simulink model "quarter_sus_imp_force"  (R2025a)
settings: Solver=FixedStepAuto  StartTime=0.0  StopTime=20  FixedStep=0.001  RelTol=1e-3
model workspace (MAT data in the model file):
  Cs : Simulink.Parameter (value not decoded)
  Cy_f1 = 128915.5
  Cy_r1 = 85943.6
  G0 : Simulink.Parameter (value not decoded)
  IDA_ISD_PBC_bd : Simulink.Parameter (value not decoded)
  IDA_ISD_PBC_c1 : Simulink.Parameter (value not decoded)
  IDA_ISD_PBC_k1 : Simulink.Parameter (value not decoded)
  IDA_ISD_PBC_k2 : Simulink.Parameter (value not decoded)
  IDA_ISD_PBC_r1 : Simulink.Parameter (value not decoded)
  IDA_PBC_cd4 = 2000
  IDA_PBC_kd2 = 10000
  IDA_PBC_r1 = 1.5
  IDA_PBC_r2 = 0.44
  ISD_1_b : Simulink.Parameter (value not decoded)
  ISD_1_c : Simulink.Parameter (value not decoded)
  ISD_1_k1 : Simulink.Parameter (value not decoded)
  ISD_1_k2 : Simulink.Parameter (value not decoded)
  Izz1 = 1536.7
  Ks : Simulink.Parameter (value not decoded)
  Kt : Simulink.Parameter (value not decoded)
  Q : Simulink.Parameter (value not decoded)
  Q_F : Simulink.Parameter (value not decoded)
  Q_b_deflec : Simulink.Parameter (value not decoded)
  Q_delta_F : Simulink.Parameter (value not decoded)
  Q_dot : Simulink.Parameter (value not decoded)
  Q_dot_s : Simulink.Parameter (value not decoded)
  Q_dot_s_h : Simulink.Parameter (value not decoded)
  Q_dot_u : Simulink.Parameter (value not decoded)
  Q_flec : Simulink.Parameter (value not decoded)
  Q_flec_t : Simulink.Parameter (value not decoded)
  SHADD_alpha : Simulink.Parameter (value not decoded)
  a1 = 1.015
  a_max : Simulink.Parameter (value not decoded)
  a_min : Simulink.Parameter (value not decoded)
  adva_max : Simulink.Parameter (value not decoded)
  adva_min : Simulink.Parameter (value not decoded)
  as_max : Simulink.Parameter (value not decoded)
  b1 = 1.895
  b_deflec : Simulink.Parameter (value not decoded)
  bump_height : Simulink.Parameter (value not decoded)
  bump_lenth : Simulink.Parameter (value not decoded)
  bump_start : Simulink.Parameter (value not decoded)
  damper_param : Simulink.Parameter (value not decoded)
  deflec_max : Simulink.Parameter (value not decoded)
  done_range : Simulink.Parameter (value not decoded)
  f0 : Simulink.Parameter (value not decoded)
  h1 = 0.54
  imp_Cs : Simulink.Parameter (value not decoded)
  imp_Ks : Simulink.Parameter (value not decoded)
  imp_Ms : Simulink.Parameter (value not decoded)
  inerter_b : Simulink.Parameter (value not decoded)
  inerter_b_2 : Simulink.Parameter (value not decoded)
  inerter_c : Simulink.Parameter (value not decoded)
  inerter_k : Simulink.Parameter (value not decoded)
  inerter_k_2 : Simulink.Parameter (value not decoded)
  ms : Simulink.Parameter (value not decoded)
  mu : Simulink.Parameter (value not decoded)
  noise_seed : Simulink.Parameter (value not decoded)
  omega_1 : Simulink.Parameter (value not decoded)
  omega_2 : Simulink.Parameter (value not decoded)
  omega_3 : Simulink.Parameter (value not decoded)
  omega_4 : Simulink.Parameter (value not decoded)
  omega_5 : Simulink.Parameter (value not decoded)
  punish_Q : Simulink.Parameter (value not decoded)
  punish_R : Simulink.Parameter (value not decoded)
  reward_w_as : Simulink.Parameter (value not decoded)
  reward_w_au : Simulink.Parameter (value not decoded)
  reward_w_defv : Simulink.Parameter (value not decoded)
  road_seed : Simulink.Parameter (value not decoded)
  road_type : Simulink.Parameter (value not decoded)
  sigma_f1 = 0.1
  sigma_r1 = 0.1
  sine_amp : Simulink.Parameter (value not decoded)
  sine_freq : Simulink.Parameter (value not decoded)
  u : Simulink.Parameter (value not decoded)
  vs0 : Simulink.Parameter (value not decoded)
  vu0 : Simulink.Parameter (value not decoded)
  x_max : Simulink.Parameter (value not decoded)
  x_min : Simulink.Parameter (value not decoded)
  xs0 : Simulink.Parameter (value not decoded)
  xu0 : Simulink.Parameter (value not decoded)
symbols that are objects in the model workspace (value not decoded): a_max, a_min, b_deflec, bump_height, bump_lenth, bump_start, Cs, damper_param, f0, G0, IDA_ISD_PBC_bd, IDA_ISD_PBC_c1, IDA_ISD_PBC_k1, IDA_ISD_PBC_k2, IDA_ISD_PBC_r1, imp_Cs, imp_Ks, imp_Ms, Ks, Kt, ms, mu, omega_1, omega_2, omega_3, omega_4, omega_5, Q_b_deflec, Q_delta_F, Q_dot_s, Q_dot_s_h, Q_dot_u, Q_F, Q_flec, Q_flec_t, road_type, SHADD_alpha, sine_amp, sine_freq, vs0, vu0, xs0, xu0
undefined symbols (not defined in the file): ADD, Force, IDA, Imp, Imp_Force, PBC, SH, Train, Validation
libraries: fl_lib x32, nesl_utility x27, sharedTrackingLibrary x4, sdl_lib x2, dspstat3 x2, deeplib x1, simulink x1
(part 6 of 6)

== system quarter_sus_imp_force/QuarterSuspension /Variant Subsystem/Train-Imp_Force/Subsystem/MATLAB Function2/EKF epsilon ==
  y : Inport
  epsilon : Inport  Port=2
  Constant : Constant  Value=diag([0,0,1,0])
  Constant7 : Constant  Value=500  SampleTime=0.001
  Extended Kalman Filter1 : sharedTrackingLibrary/Extended Kalman Filter  StateTransitionFcn=IFEKF_tfcn_ep  HasStateTransitionJacobianFcn=on  StateTransitionJacobianFcn=IFEKF_jcob_fcn_ep  HasAdditiveProcessNoise=Additive  ProcessNoise=[0,0,1e-7,1e-10]  HasTimeVaryingProcessNoise=on  HasStateTransitionFcnExtraArgument=1  InitialState=[0;-0.2;1*2*pi;0.2;]  InitialStateCovariance=[1e-1,1e-1,1e-1,1e-5]  MeasurementFcn1=IFEKF_measure_fcn_mod  HasMeasurementJacobianFcn1=on  MeasurementJacobianFcn1=IFEKF_mea_jcob_fcn_mod  HasMeasurementEnablePort1=off  HasAdditiveMeasurementNoise1=Additive  MeasurementNoise1=0.0001  HasTimeVaryingMeasurementNoise1=on  HasMeasurementFcnExtraArgument1=0  HasMeasurementWrapping1=off  MeasurementFcn2=myMeasurementFcn  HasMeasurementJacobianFcn2=off  HasMeasurementEnablePort2=off  HasAdditiveMeasurementNoise2=Additive  MeasurementNoise2=1  HasTimeVaryingMeasurementNoise2=off  HasMeasurementFcnExtraArgument2=0  HasMeasurementWrapping2=off  MeasurementFcn3=myMeasurementFcn  HasMeasurementJacobianFcn3=off  HasMeasurementEnablePort3=off  HasAdditiveMeasurementNoise3=Additive  MeasurementNoise3=1  HasTimeVaryingMeasurementNoise3=off  HasMeasurementFcnExtraArgument3=0  HasMeasurementWrapping3=off  MeasurementFcn4=myMeasurementFcn  HasMeasurementJacobianFcn4=off  HasMeasurementEnablePort4=off  HasAdditiveMeasurementNoise4=Additive  MeasurementNoise4=1  HasTimeVaryingMeasurementNoise4=off  HasMeasurementFcnExtraArgument4=0  HasMeasurementWrapping4=off  MeasurementFcn5=myMeasurementFcn  HasMeasurementJacobianFcn5=off  HasMeasurementEnablePort5=off  HasAdditiveMeasurementNoise5=Additive  MeasurementNoise5=1  HasTimeVaryingMeasurementNoise5=off  HasMeasurementFcnExtraArgument5=0  HasMeasurementWrapping5=off  EnableMultirate=off  StateTransitionFcnSampleTime=1  MeasurementFcn1SampleTime=1  MeasurementFcn2SampleTime=1  MeasurementFcn3SampleTime=1  MeasurementFcn4SampleTime=1  MeasurementFcn5SampleTime=1  UseCurrentEstimator=off  OutputStateCovariance=on  DataType=double  SampleTime=0.001  NumberOfMeasurements=1
  Gain6 : Gain  Gain=1/2/pi
  Scope6 : Scope
      settings: ActiveDisplayYMinimum=-0.3996  ActiveDisplayYMaximum=6.537  DataLoggingVariableName=ScopeData2
  Selector1 : Selector  InputPortWidth=4  IndexOptions=Index vector (dialog)  Indices=[1]  OutputSizes=1
  Selector8 : Selector  InputPortWidth=4  IndexOptions=Index vector (dialog)  Indices=[3]  OutputSizes=1
  x1hat : Outport
  P : Outport  Port=2
  debug : Outport  Port=3
  xhat_pred : Outport  Port=4
  y_residual : Outport  Port=5
  omega : Outport  Port=6
  wires:
  y/1 -> Extended Kalman Filter1/3
  Extended Kalman Filter1/2 -> P/1
  Constant7/1 -> Extended Kalman Filter1/4
  epsilon/1 -> Extended Kalman Filter1/2
  Constant/1 -> Extended Kalman Filter1/1
  Gain6/1 -> omega/1, Scope6/1
  Selector8/1 -> Gain6/1
  Extended Kalman Filter1/1 -> Selector1/1, Selector8/1
  Selector1/1 -> x1hat/1

== system quarter_sus_imp_force/QuarterSuspension /Variant Subsystem/Train-Imp_Force/Subsystem/MATLAB Function2/EKF simple Amp ==
  y : Inport
  epsilon : Inport  Port=2
  Constant5 : Constant  Value=0.1e-5
  Constant7 : Constant  Value=0.11  SampleTime=0.001
  Extended Kalman Filter1 : sharedTrackingLibrary/Extended Kalman Filter  StateTransitionFcn=IFEKF_tfcn_amp  HasStateTransitionJacobianFcn=on  StateTransitionJacobianFcn=IFEKF_jcob_fcn_amp  HasAdditiveProcessNoise=Additive  ProcessNoise=[0,0,1e-7,1e-10]  HasTimeVaryingProcessNoise=on  HasStateTransitionFcnExtraArgument=1  InitialState=[0;-0.5;2*pi;0.5;]  InitialStateCovariance=[1e-1,1e-1,1e-1,1e-5]  MeasurementFcn1=IFEKF_measure_fcn_amp  HasMeasurementJacobianFcn1=on  MeasurementJacobianFcn1=IFEKF_mea_jcob_fcn_amp  HasMeasurementEnablePort1=off  HasAdditiveMeasurementNoise1=Additive  MeasurementNoise1=0.0001  HasTimeVaryingMeasurementNoise1=on  HasMeasurementFcnExtraArgument1=0  HasMeasurementWrapping1=off  MeasurementFcn2=myMeasurementFcn  HasMeasurementJacobianFcn2=off  HasMeasurementEnablePort2=off  HasAdditiveMeasurementNoise2=Additive  MeasurementNoise2=1  HasTimeVaryingMeasurementNoise2=off  HasMeasurementFcnExtraArgument2=0  HasMeasurementWrapping2=off  MeasurementFcn3=myMeasurementFcn  HasMeasurementJacobianFcn3=off  HasMeasurementEnablePort3=off  HasAdditiveMeasurementNoise3=Additive  MeasurementNoise3=1  HasTimeVaryingMeasurementNoise3=off  HasMeasurementFcnExtraArgument3=0  HasMeasurementWrapping3=off  MeasurementFcn4=myMeasurementFcn  HasMeasurementJacobianFcn4=off  HasMeasurementEnablePort4=off  HasAdditiveMeasurementNoise4=Additive  MeasurementNoise4=1  HasTimeVaryingMeasurementNoise4=off  HasMeasurementFcnExtraArgument4=0  HasMeasurementWrapping4=off  MeasurementFcn5=myMeasurementFcn  HasMeasurementJacobianFcn5=off  HasMeasurementEnablePort5=off  HasAdditiveMeasurementNoise5=Additive  MeasurementNoise5=1  HasTimeVaryingMeasurementNoise5=off  HasMeasurementFcnExtraArgument5=0  HasMeasurementWrapping5=off  EnableMultirate=off  StateTransitionFcnSampleTime=1  MeasurementFcn1SampleTime=1  MeasurementFcn2SampleTime=1  MeasurementFcn3SampleTime=1  MeasurementFcn4SampleTime=1  MeasurementFcn5SampleTime=1  UseCurrentEstimator=off  OutputStateCovariance=on  DataType=double  SampleTime=0.001  NumberOfMeasurements=1
  Gain6 : Gain  Gain=1/2/pi
  MATLAB Function : MATLAB Function
  Scope1 : Scope
      settings: ActiveDisplayYMinimum=-1.3479  ActiveDisplayYMaximum=7.1311  DataLoggingVariableName=ScopeData7
  Scope6 : Scope
      settings: ActiveDisplayYMinimum=0.95  ActiveDisplayYMaximum=1.05
  Selector1 : Selector  InputPortWidth=4  IndexOptions=Index vector (dialog)  Indices=[1]  OutputSizes=1
  Selector8 : Selector  InputPortWidth=4  IndexOptions=Index vector (dialog)  Indices=[3]  OutputSizes=1
  x1hat : Outport
  P : Outport  Port=2
  debug : Outport  Port=3
  xhat_pred : Outport  Port=4
  y_residual : Outport  Port=5
  omega : Outport  Port=6
  wires:
  epsilon/1 -> Extended Kalman Filter1/2
  Constant7/1 -> Extended Kalman Filter1/4
  Constant5/1 -> MATLAB Function/1(gamma)
  Extended Kalman Filter1/2 -> P/1
  y/1 -> Extended Kalman Filter1/3
  MATLAB Function/1(y) -> Extended Kalman Filter1/1
  Extended Kalman Filter1/1 -> Selector1/1, Selector8/1, Scope1/1
  Selector8/1 -> Gain6/1
  Gain6/1 -> omega/1, Scope6/1
  Selector1/1 -> x1hat/1

== system quarter_sus_imp_force/QuarterSuspension /Variant Subsystem/Train-Imp_Force/Subsystem/MATLAB Function2/IFEKF simple ==
  y : Inport
  Constant : Constant  Value=diag([0,0,0,0,1])
  Constant7 : Constant  Value=10  SampleTime=0.001
  Extended Kalman Filter1 : sharedTrackingLibrary/Extended Kalman Filter  StateTransitionFcn=IFEKF_tfcn_simp  HasStateTransitionJacobianFcn=on  StateTransitionJacobianFcn=IFEKF_jcob_fcn_simp  HasAdditiveProcessNoise=Additive  ProcessNoise=[0,0,1e-7,1e-10,0]  HasTimeVaryingProcessNoise=on  HasStateTransitionFcnExtraArgument=0  InitialState=[0;-1;0;-1;0.1*pi;]  InitialStateCovariance=[1e-1,1e-1,1e-1,1e-1,1e-5]  MeasurementFcn1=IFEKF_measure_fcn_simp  HasMeasurementJacobianFcn1=on  MeasurementJacobianFcn1=IFEKF_mea_jcob_fcn_simp  HasMeasurementEnablePort1=off  HasAdditiveMeasurementNoise1=Additive  MeasurementNoise1=0.0001  HasTimeVaryingMeasurementNoise1=on  HasMeasurementFcnExtraArgument1=0  HasMeasurementWrapping1=off  MeasurementFcn2=myMeasurementFcn  HasMeasurementJacobianFcn2=off  HasMeasurementEnablePort2=off  HasAdditiveMeasurementNoise2=Additive  MeasurementNoise2=1  HasTimeVaryingMeasurementNoise2=off  HasMeasurementFcnExtraArgument2=0  HasMeasurementWrapping2=off  MeasurementFcn3=myMeasurementFcn  HasMeasurementJacobianFcn3=off  HasMeasurementEnablePort3=off  HasAdditiveMeasurementNoise3=Additive  MeasurementNoise3=1  HasTimeVaryingMeasurementNoise3=off  HasMeasurementFcnExtraArgument3=0  HasMeasurementWrapping3=off  MeasurementFcn4=myMeasurementFcn  HasMeasurementJacobianFcn4=off  HasMeasurementEnablePort4=off  HasAdditiveMeasurementNoise4=Additive  MeasurementNoise4=1  HasTimeVaryingMeasurementNoise4=off  HasMeasurementFcnExtraArgument4=0  HasMeasurementWrapping4=off  MeasurementFcn5=myMeasurementFcn  HasMeasurementJacobianFcn5=off  HasMeasurementEnablePort5=off  HasAdditiveMeasurementNoise5=Additive  MeasurementNoise5=1  HasTimeVaryingMeasurementNoise5=off  HasMeasurementFcnExtraArgument5=0  HasMeasurementWrapping5=off  EnableMultirate=off  StateTransitionFcnSampleTime=1  MeasurementFcn1SampleTime=1  MeasurementFcn2SampleTime=1  MeasurementFcn3SampleTime=1  MeasurementFcn4SampleTime=1  MeasurementFcn5SampleTime=1  UseCurrentEstimator=off  OutputStateCovariance=on  DataType=double  SampleTime=0.001  NumberOfMeasurements=1
  Gain6 : Gain  Gain=1/2/pi
  Scope1 : Scope
      settings: ActiveDisplayYMinimum=-108223.313  ActiveDisplayYMaximum=120159.3313  DataLoggingVariableName=ScopeData2
  Scope6 : Scope
      settings: ActiveDisplayYMinimum=-5.0452  ActiveDisplayYMaximum=3.9569  DataLoggingVariableName=ScopeData3
  Selector1 : Selector  InputPortWidth=5  IndexOptions=Index vector (dialog)  Indices=[1]  OutputSizes=1
  Selector8 : Selector  InputPortWidth=5  IndexOptions=Index vector (dialog)  Indices=[5]  OutputSizes=1
  x1hat : Outport
  P : Outport  Port=2
  debug : Outport  Port=3
  xhat_pred : Outport  Port=4
  y_residual : Outport  Port=5
  omega : Outport  Port=6
  wires:
  y/1 -> Extended Kalman Filter1/2
  Extended Kalman Filter1/2 -> P/1
  Constant7/1 -> Extended Kalman Filter1/3
  Constant/1 -> Extended Kalman Filter1/1
  Gain6/1 -> omega/1, Scope6/1
  Selector8/1 -> Gain6/1
  Selector1/1 -> x1hat/1
  Extended Kalman Filter1/1 -> Selector1/1, Selector8/1, Scope1/1

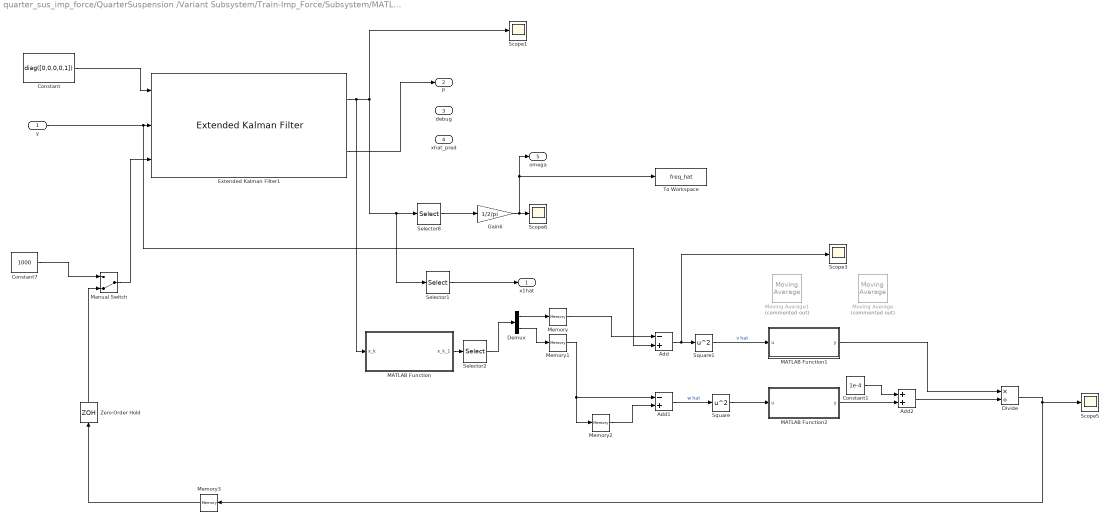
== system quarter_sus_imp_force/QuarterSuspension /Variant Subsystem/Train-Imp_Force/Subsystem/MATLAB Function2/adaptive IFEKF simple ==
  y : Inport
  Add : Sum  Inputs=-+
  Add1 : Sum  Inputs=-+
  Add2 : Sum
  Constant : Constant  Value=diag([0,0,0,0,1])
  Constant1 : Constant  Value=1e-4
  Constant7 : Constant  Value=1000  SampleTime=0.001
  Demux : Demux  Outputs=2
  Divide : Product  Inputs=*/
  Extended Kalman Filter1 : sharedTrackingLibrary/Extended Kalman Filter  StateTransitionFcn=IFEKF_tfcn_simp  HasStateTransitionJacobianFcn=on  StateTransitionJacobianFcn=IFEKF_jcob_fcn_simp  HasAdditiveProcessNoise=Additive  ProcessNoise=[0,0,1e-7,1e-10,0]  HasTimeVaryingProcessNoise=on  HasStateTransitionFcnExtraArgument=0  InitialState=[0;-1;0;-1;0.1*pi;]  InitialStateCovariance=[1e-1,1e-1,1e-1,1e-1,1e-5]  MeasurementFcn1=IFEKF_measure_fcn_simp  HasMeasurementJacobianFcn1=on  MeasurementJacobianFcn1=IFEKF_mea_jcob_fcn_simp  HasMeasurementEnablePort1=off  HasAdditiveMeasurementNoise1=Additive  MeasurementNoise1=0.0001  HasTimeVaryingMeasurementNoise1=on  HasMeasurementFcnExtraArgument1=0  HasMeasurementWrapping1=off  MeasurementFcn2=myMeasurementFcn  HasMeasurementJacobianFcn2=off  HasMeasurementEnablePort2=off  HasAdditiveMeasurementNoise2=Additive  MeasurementNoise2=1  HasTimeVaryingMeasurementNoise2=off  HasMeasurementFcnExtraArgument2=0  HasMeasurementWrapping2=off  MeasurementFcn3=myMeasurementFcn  HasMeasurementJacobianFcn3=off  HasMeasurementEnablePort3=off  HasAdditiveMeasurementNoise3=Additive  MeasurementNoise3=1  HasTimeVaryingMeasurementNoise3=off  HasMeasurementFcnExtraArgument3=0  HasMeasurementWrapping3=off  MeasurementFcn4=myMeasurementFcn  HasMeasurementJacobianFcn4=off  HasMeasurementEnablePort4=off  HasAdditiveMeasurementNoise4=Additive  MeasurementNoise4=1  HasTimeVaryingMeasurementNoise4=off  HasMeasurementFcnExtraArgument4=0  HasMeasurementWrapping4=off  MeasurementFcn5=myMeasurementFcn  HasMeasurementJacobianFcn5=off  HasMeasurementEnablePort5=off  HasAdditiveMeasurementNoise5=Additive  MeasurementNoise5=1  HasTimeVaryingMeasurementNoise5=off  HasMeasurementFcnExtraArgument5=0  HasMeasurementWrapping5=off  EnableMultirate=off  StateTransitionFcnSampleTime=1  MeasurementFcn1SampleTime=1  MeasurementFcn2SampleTime=1  MeasurementFcn3SampleTime=1  MeasurementFcn4SampleTime=1  MeasurementFcn5SampleTime=1  UseCurrentEstimator=off  OutputStateCovariance=on  DataType=double  SampleTime=0.001  NumberOfMeasurements=1
  Gain6 : Gain  Gain=1/2/pi
  MATLAB Function : MATLAB Function  TreatAsAtomicUnit=on
  MATLAB Function1 : MATLAB Function  TreatAsAtomicUnit=on
  MATLAB Function2 : MATLAB Function  TreatAsAtomicUnit=on
  Manual Switch : ManualSwitch  CurrentSetting=0
  Memory : Memory  InitialCondition=5
  Memory1 : Memory
  Memory2 : Memory  InitialCondition=1
  Memory3 : Memory  InitialCondition=10
  Moving Average : dspstat3/Moving Average  Commented=on  Method=Exponential weighting  ForgettingFactorPort=off  SpecifyWindowLength=off  WindowLength=100  OverlapLength=50  AllowArbitraryInputLength=on  ForgettingFactor=0.999  SimulateUsing=Interpreted execution
  Moving Average1 : dspstat3/Moving Average  Commented=on  Method=Sliding window  ForgettingFactorPort=off  SpecifyWindowLength=off  WindowLength=100  OverlapLength=50  AllowArbitraryInputLength=off  ForgettingFactor=0.999  SimulateUsing=Code generation
  Scope{1,3,5..6} (4 alike) : Scope
      Scope1 settings: ActiveDisplayYMinimum=-5.9836760801118811E+37  ActiveDisplayYMaximum=5.3206752918754988E+37  DataLoggingVariableName=ScopeData3
      Scope3 settings: ActiveDisplayYMinimum=-5.9322  ActiveDisplayYMaximum=3.4471  DataLoggingVariableName=ScopeData4
      Scope5 settings: ActiveDisplayYMinimum=-182.5988  ActiveDisplayYMaximum=1643.3904  DataLoggingVariableName=ScopeData6
      Scope6 settings: ActiveDisplayYMinimum=-3.1891  ActiveDisplayYMaximum=3.1646  DataLoggingVariableName=ScopeData8
  Selector1 : Selector  InputPortWidth=5  IndexOptions=Index vector (dialog)  Indices=[1]  OutputSizes=1
  Selector2 : Selector  InputPortWidth=5  IndexOptions=Index vector (dialog)  Indices=[1 5]  OutputSizes=1
  Selector8 : Selector  InputPortWidth=5  IndexOptions=Index vector (dialog)  Indices=[5]  OutputSizes=1
  Square : Math  Operator=square
  Square1 : Math  Operator=square
  To Workspace : ToWorkspace  VariableName=freq_hat  SampleTime=-1
  Zero-Order Hold : ZeroOrderHold  SampleTime=0.001
  x1hat : Outport
  P : Outport  Port=2
  debug : Outport  Port=3
  xhat_pred : Outport  Port=4
  omega : Outport  Port=5
  wires:
  Add1/1 -> Square/1  "w hat"
  Demux/2 -> Memory1/1
  Constant1/1 -> Add2/1
  Zero-Order Hold/1 -> Manual Switch/2
  Memory2/1 -> Add1/2
  Manual Switch/1 -> Extended Kalman Filter1/3
  MATLAB Function/1(x_k_1) -> Selector2/1
  MATLAB Function1/1(y) -> Divide/1
  Selector2/1 -> Demux/1
  Add2/1 -> Divide/2
  Constant/1 -> Extended Kalman Filter1/1
  Selector1/1 -> x1hat/1
  MATLAB Function2/1(y) -> Add2/2
  Memory/1 -> Add/1
  Extended Kalman Filter1/1 -> MATLAB Function/1(x_k), Scope1/1, Selector8/1, Selector1/1
  y/1 -> Add/2, Extended Kalman Filter1/2
  Memory1/1 -> Add1/1, Memory2/1
  Square/1 -> MATLAB Function2/1(u)
  Square1/1 -> MATLAB Function1/1(u)  "v hat"
  Extended Kalman Filter1/2 -> P/1
  Divide/1 -> Memory3/1, Scope5/1
  Selector8/1 -> Gain6/1
  Demux/1 -> Memory/1
  Add/1 -> Scope3/1, Square1/1
  Memory3/1 -> Zero-Order Hold/1
  Gain6/1 -> Scope6/1, To Workspace/1, omega/1
  Constant7/1 -> Manual Switch/1

== matlab function quarter_sus_imp_force/QuarterSuspension /Variant Subsystem/IDA-PBC/Subsystem/我的控制/MATLAB Function ==
  data: cs input; ks input; ct input; r1 input; u output; r2 input; kd2 input; cd4 input; q1 input; q2 input; dq1 input; dq2 input
function u = calculateEquation(cs, ks,ct, r1, r2, kd2,cd4, q1,q2,dq1,dq2)
    % Calculate each term of the equation
    term1 = (ks - r2*kd2)*q1;
    term2 = (r1 - r2)*kd2*q2 + cs*dq1;
    % term4 = r2 * (r2 - r1)* cd4;
    term3 = (cd4/2 - cd4/r2 + (2*cd4)/(-r1 + r2)+cs)*dq1;
    
    term5 = (cd4/2 - (cd4*r1)/(2*r2)) * dq2;

    % Sum all terms to get u
    u = term1 + term2 + term3 - term5;
end

== matlab function quarter_sus_imp_force/QuarterSuspension /Variant Subsystem/PDD/Subsystem1/MATLAB Function ==
  data: Kxsvs input; y output; cmax input; cmin input; vdef input; xdef input; Cs input
function y = PDD_switch(Kxsvs,cmax,cmin,vdef, xdef,Cs)
vdef2 = vdef^2;
    if (Kxsvs + ((cmax + Cs) * vdef2)) < 0
        y = 1;
    elseif (vdef == 0) && (xdef ~= 0) 
        y = 3;
    elseif (Kxsvs + ((cmin +Cs) *vdef2)) >= 0
        y = 2;
    else
        y = 4 ;
    end
end

== matlab function quarter_sus_imp_force/QuarterSuspension /Variant Subsystem/IDA-PBC/Subsystem/IDA-PBC 论文控制/MATLAB Function ==
  data: cs input; ks input; ct input; r1 input; u output; r2 input; kd2 input; cd4 input; q1 input; q2 input; dq1 input; dq2 input
function u = calculateEquation(cs, ks,ct, r1, r2, kd2,cd4, q1,q2,dq1,dq2)
    % Calculate each term of the equation
    term1 = (ks - r2*kd2)*q1;
    term2 = (r1 - r2)*kd2*q2 + cs*dq1;
    term4 = r2 * (r2 - r1)* cd4;
    term3 = ((r1*r2*(r2 - 2)*ct +term4)*dq1) / (r1 - r2)^2;
    
    term5 = (ct*r1*r2 / (r1 - r2) - cd4) * dq2;

    % Sum all terms to get u
    u = term1 + term2 + term3 - term5;
end

== matlab function quarter_sus_imp_force/QuarterSuspension /Subsystem1/Semi Active Suspension/Damper/Hysteretic/MATLAB Function1 ==
  data: displacement input; F_d output; velocity input; I input; params input
function F_d = improvedHystereticModel(displacement, velocity, I, params)
    % 从params数组中提取模型参数
    c1 = params(1); c2 = params(2); c3 = params(3);
    k1 = params(4); k2 = params(5); k3 = params(6);
    alpha1 = params(7); alpha2 = params(8);
    % f01 = params(9); f02 = params(10); f03 = params(11); % 这些参数似乎在模型中未使用
    gamma1 = params(12); gamma2 = params(13); gamma3 = params(14);
    beta = params(15); delta = params(16);

    % 根据I计算c, k, alpha, 和 gamma
    c = c1 * I^2 + c2 * I + c3;
    k = k1 * I^2 + k2 * I + k3;
    alpha = alpha1 * I + alpha2;
    gamma = gamma1 * I^2 + gamma2 * I + gamma3;

    % 计算c^*和z
    c_star = gamma * (sign(velocity) + 1);
    z = tanh(beta * velocity + delta * sign(displacement));

    % 计算减震器力
    F_d = (c + c_star) * velocity + k * displacement + alpha * z;
end

== matlab function quarter_sus_imp_force/QuarterSuspension /Subsystem1/Semi Active Suspension/Damper/Random Current/MATLAB Function1 ==
  data: displacement input; F_d output; velocity input; I input; params input
function F_d = improvedHystereticModel(displacement, velocity, I, params)
    % 从params数组中提取模型参数
    c1 = params(1); c2 = params(2); c3 = params(3);
    k1 = params(4); k2 = params(5); k3 = params(6);
    alpha1 = params(7); alpha2 = params(8);
    % f01 = params(9); f02 = params(10); f03 = params(11); % 这些参数似乎在模型中未使用
    gamma1 = params(12); gamma2 = params(13); gamma3 = params(14);
    beta = params(15); delta = params(16);

    % 根据I计算c, k, alpha, 和 gamma
    c = c1 * I^2 + c2 * I + c3;
    k = k1 * I^2 + k2 * I + k3;
    alpha = alpha1 * I + alpha2;
    gamma = gamma1 * I^2 + gamma2 * I + gamma3;

    % 计算c^*和z
    c_star = gamma * (sign(velocity) + 1);
    z = tanh(beta * velocity + delta * sign(displacement));

    % 计算减震器力
    F_d = (c + c_star) * velocity + k * displacement + alpha * z;
end

== matlab function quarter_sus_imp_force/QuarterSuspension /Subsystem1/Semi Active Suspension/Damper/semi-active/MATLAB Function1 ==
  data: displacement input; F_d output; velocity input; I input; params input
function F_d = improvedHystereticModel(displacement, velocity, I, params)
    % 从params数组中提取模型参数
    c1 = params(1); c2 = params(2); c3 = params(3);
    k1 = params(4); k2 = params(5); k3 = params(6);
    alpha1 = params(7); alpha2 = params(8);
    % f01 = params(9); f02 = params(10); f03 = params(11); % 这些参数似乎在模型中未使用
    gamma1 = params(12); gamma2 = params(13); gamma3 = params(14);
    beta = params(15); delta = params(16);

    % 根据I计算c, k, alpha, 和 gamma
    c = c1 * I^2 + c2 * I + c3;
    k = k1 * I^2 + k2 * I + k3;
    alpha = alpha1 * I + alpha2;
    gamma = gamma1 * I^2 + gamma2 * I + gamma3;

    % 计算c^*和z
    c_star = gamma * (sign(velocity) + 1);
    z = tanh(beta * velocity + delta * sign(displacement));

    % 计算减震器力
    F_d = (c + c_star) * velocity + k * displacement + alpha * z;
end

== matlab function quarter_sus_imp_force/QuarterSuspension /Variant Subsystem/IDA-PBC/Subsystem/IDA_ISD_1号参考控制/MATLAB Function ==
  data: cs input; ks input; ct input; r1 input; u output; r2 input; k1 input; k2 input; c1 input; q1 input; q2 input; dq1 input; xs input; dxs input; xb input; dxb input
function u = calculateEquation(cs, ks,ct, r1, r2,k1, k2,c1, q1,q2,dq1,xs,dxs,xb,dxb)
    % Calculate each term of the equation
  
    term1 = ks*q1;
    term2 = (cs+c1)*dq1;

    term4 = -k2*(xs-xb)/r1;

    term3 = -k1*q2/r1;
    
    term5 = -c1*(dxs-dxb);

    % Sum all terms to get u
    u = term1 + term2 + term3 +term4+ term5;
end

== matlab function quarter_sus_imp_force/QuarterSuspension /Variant Subsystem/IDA-PBC/Subsystem/IDA_ISD_1号参考控制/virtual Inerter/MATLAB Function ==
  data: as input; y output; xu input; vu input; xb input; vb input; k1 input; c1 input; bd input
function y = fcn(as,xu,vu,xb,vb,k1,c1,bd)

y = as-(k1*(xb-xu)+c1*(vb-vu))/bd;

== matlab function quarter_sus_imp_force/QuarterSuspension /Subsystem1/Semi Active Air Suspension simscape/Damper/Hysteretic/MATLAB Function1 ==
  data: displacement input; F_d output; velocity input; I input; params input
function F_d = improvedHystereticModel(displacement, velocity, I, params)
    % 从params数组中提取模型参数
    c1 = params(1); c2 = params(2); c3 = params(3);
    k1 = params(4); k2 = params(5); k3 = params(6);
    alpha1 = params(7); alpha2 = params(8);
    % f01 = params(9); f02 = params(10); f03 = params(11); % 这些参数似乎在模型中未使用
    gamma1 = params(12); gamma2 = params(13); gamma3 = params(14);
    beta = params(15); delta = params(16);

    % 根据I计算c, k, alpha, 和 gamma
    c = c1 * I^2 + c2 * I + c3;
    k = k1 * I^2 + k2 * I + k3;
    alpha = alpha1 * I + alpha2;
    gamma = gamma1 * I^2 + gamma2 * I + gamma3;

    % 计算c^*和z
    c_star = gamma * (sign(velocity) + 1);
    z = tanh(beta * velocity + delta * sign(displacement));

    % 计算减震器力
    F_d = (c + c_star) * velocity + k * displacement + alpha * z;
end

== matlab function quarter_sus_imp_force/QuarterSuspension /Subsystem1/Semi Active Air Suspension simscape/Damper/Random Current/MATLAB Function1 ==
  data: displacement input; F_d output; velocity input; I input; params input
function F_d = improvedHystereticModel(displacement, velocity, I, params)
    % 从params数组中提取模型参数
    c1 = params(1); c2 = params(2); c3 = params(3);
    k1 = params(4); k2 = params(5); k3 = params(6);
    alpha1 = params(7); alpha2 = params(8);
    % f01 = params(9); f02 = params(10); f03 = params(11); % 这些参数似乎在模型中未使用
    gamma1 = params(12); gamma2 = params(13); gamma3 = params(14);
    beta = params(15); delta = params(16);

    % 根据I计算c, k, alpha, 和 gamma
    c = c1 * I^2 + c2 * I + c3;
    k = k1 * I^2 + k2 * I + k3;
    alpha = alpha1 * I + alpha2;
    gamma = gamma1 * I^2 + gamma2 * I + gamma3;

    % 计算c^*和z
    c_star = gamma * (sign(velocity) + 1);
    z = tanh(beta * velocity + delta * sign(displacement));

    % 计算减震器力
    F_d = (c + c_star) * velocity + k * displacement + alpha * z;
end

== matlab function quarter_sus_imp_force/QuarterSuspension /Subsystem1/Semi Active Air Suspension simscape/Damper/semi-active/MATLAB Function1 ==
  data: displacement input; F_d output; velocity input; I input; params input
function F_d = improvedHystereticModel(displacement, velocity, I, params)
    % 从params数组中提取模型参数
    c1 = params(1); c2 = params(2); c3 = params(3);
    k1 = params(4); k2 = params(5); k3 = params(6);
    alpha1 = params(7); alpha2 = params(8);
    % f01 = params(9); f02 = params(10); f03 = params(11); % 这些参数似乎在模型中未使用
    gamma1 = params(12); gamma2 = params(13); gamma3 = params(14);
    beta = params(15); delta = params(16);

    % 根据I计算c, k, alpha, 和 gamma
    c = c1 * I^2 + c2 * I + c3;
    k = k1 * I^2 + k2 * I + k3;
    alpha = alpha1 * I + alpha2;
    gamma = gamma1 * I^2 + gamma2 * I + gamma3;

    % 计算c^*和z
    c_star = gamma * (sign(velocity) + 1);
    z = tanh(beta * velocity + delta * sign(displacement));

    % 计算减震器力
    F_d = (c + c_star) * velocity + k * displacement + alpha * z;
end

== matlab function quarter_sus_imp_force/QuarterSuspension /Subsystem1/Semi Active Air Suspension/Damper/Hysteretic/MATLAB Function1 ==
  data: displacement input; F_d output; velocity input; I input; params input
function F_d = improvedHystereticModel(displacement, velocity, I, params)
    % 从params数组中提取模型参数
    c1 = params(1); c2 = params(2); c3 = params(3);
    k1 = params(4); k2 = params(5); k3 = params(6);
    alpha1 = params(7); alpha2 = params(8);
    % f01 = params(9); f02 = params(10); f03 = params(11); % 这些参数似乎在模型中未使用
    gamma1 = params(12); gamma2 = params(13); gamma3 = params(14);
    beta = params(15); delta = params(16);

    % 根据I计算c, k, alpha, 和 gamma
    c = c1 * I^2 + c2 * I + c3;
    k = k1 * I^2 + k2 * I + k3;
    alpha = alpha1 * I + alpha2;
    gamma = gamma1 * I^2 + gamma2 * I + gamma3;

    % 计算c^*和z
    c_star = gamma * (sign(velocity) + 1);
    z = tanh(beta * velocity + delta * sign(displacement));

    % 计算减震器力
    F_d = (c + c_star) * velocity + k * displacement + alpha * z;
end

== matlab function quarter_sus_imp_force/QuarterSuspension /Subsystem1/Semi Active Air Suspension/Damper/Random Current/MATLAB Function1 ==
  data: displacement input; F_d output; velocity input; I input; params input
function F_d = improvedHystereticModel(displacement, velocity, I, params)
    % 从params数组中提取模型参数
    c1 = params(1); c2 = params(2); c3 = params(3);
    k1 = params(4); k2 = params(5); k3 = params(6);
    alpha1 = params(7); alpha2 = params(8);
    % f01 = params(9); f02 = params(10); f03 = params(11); % 这些参数似乎在模型中未使用
    gamma1 = params(12); gamma2 = params(13); gamma3 = params(14);
    beta = params(15); delta = params(16);

    % 根据I计算c, k, alpha, 和 gamma
    c = c1 * I^2 + c2 * I + c3;
    k = k1 * I^2 + k2 * I + k3;
    alpha = alpha1 * I + alpha2;
    gamma = gamma1 * I^2 + gamma2 * I + gamma3;

    % 计算c^*和z
    c_star = gamma * (sign(velocity) + 1);
    z = tanh(beta * velocity + delta * sign(displacement));

    % 计算减震器力
    F_d = (c + c_star) * velocity + k * displacement + alpha * z;
end

== matlab function quarter_sus_imp_force/QuarterSuspension /Subsystem1/Semi Active Air Suspension/Damper/semi-active/MATLAB Function1 ==
  data: displacement input; F_d output; velocity input; I input; params input
function F_d = improvedHystereticModel(displacement, velocity, I, params)
    % 从params数组中提取模型参数
    c1 = params(1); c2 = params(2); c3 = params(3);
    k1 = params(4); k2 = params(5); k3 = params(6);
    alpha1 = params(7); alpha2 = params(8);
    % f01 = params(9); f02 = params(10); f03 = params(11); % 这些参数似乎在模型中未使用
    gamma1 = params(12); gamma2 = params(13); gamma3 = params(14);
    beta = params(15); delta = params(16);

    % 根据I计算c, k, alpha, 和 gamma
    c = c1 * I^2 + c2 * I + c3;
    k = k1 * I^2 + k2 * I + k3;
    alpha = alpha1 * I + alpha2;
    gamma = gamma1 * I^2 + gamma2 * I + gamma3;

    % 计算c^*和z
    c_star = gamma * (sign(velocity) + 1);
    z = tanh(beta * velocity + delta * sign(displacement));

    % 计算减震器力
    F_d = (c + c_star) * velocity + k * displacement + alpha * z;
end

== stateflow chart quarter_sus_imp_force/QuarterSuspension /Variant Subsystem/Train-Imp_Force/Subsystem/Chart1 ==
  state L1
    entry:count = 0;
    level = 1;
    during:count = count+1;
    level = 1;
  state L2
    entry:count = 0;
    level = 2;
    during:count = count+1;
    level = 2;
  state L3
    entry:count = 0;
    level = 3;
    during:count = count+1;
    level = 3;
  state L4
    entry:count = 0;
    level = 4;
    during:count = count+1;
    level = 4;
  state L5
    entry:count = 0;
    level = 5;
    during:count = count+1;
    level = 5;
  state L6
    entry:count = 0;
    level = 6;
    during:count = count+1;
    level = 6;
  state L7
    entry:count = 0;
    level = 7;
    during:count = count+1;
    level = 7;
  (default) -> L1
  L1 -> L2 : [freq > (FS1+0.1)&&freq < (FS2-0.1)&&count>=200]
  L6 -> L7 [order 2] : [freq > (FS6+0.1)&&count>=100]
  L2 -> L1 [order 2] : [(freq<(FS1-0.1)&&count>=200)]
  L2 -> L3 [order 1] : [freq > (FS2+0.1)&&freq<(FS3-0.1)&&count>=100]
  L3 -> L4 [order 1] : [freq > (FS3+0.1)&&freq<(FS4-0.1)&&count>=100]
  L4 -> L5 [order 1] : [freq > (FS4+0.1)&&freq<(FS5-0.1)&&count>=100]
  L5 -> L6 [order 2] : [freq > (FS5+0.1)&&freq<(FS6-0.1)&&count>=100]
  L3 -> L2 [order 2] : [freq > (FS1+0.1)&&freq < (FS2-0.1)&&count>=100]
  L7 -> L6 : [freq > (FS5+0.1)&&freq<(FS6-0.1)&&count>=100]
  L5 -> L4 [order 1] : [freq > (FS3+0.1)&&freq<(FS4-0.1)&&count>=100]
  L6 -> L5 [order 1] : [freq > (FS4+0.1)&&freq<(FS5-0.1)&&count>=100]
  L4 -> L3 [order 2] : [freq > (FS2+0.1)&&freq<(FS3-0.1)&&count>=100]
  data: freq input; level output; FS3 constant double =7; count local; FS1 constant double =0.85; FS2 constant double =2.6; FS4 constant double =10; FS5 constant double =12.3; FS6 constant double =13.9

== matlab function quarter_sus_imp_force/QuarterSuspension /Variant Subsystem/Train-Imp_Force/Subsystem/MATLAB Function2/EKF simple Amp/MATLAB Function ==
  data: gamma input; y output size=[4,4]
function y = fcn(gamma)
% u = [0;0;gamma;1];
u = [0;0;1;gamma];
y = diag(u);
end

== matlab function quarter_sus_imp_force/QuarterSuspension /Variant Subsystem/Train-Imp_Force/Subsystem/MATLAB Function2/adaptive IFEKF simple/MATLAB Function ==
  data: x_k input; x_k_1 output
function x_k_1 = IFEKF_tfcn_simp(x_k)
x_k_1 = zeros(5,1);
dt = 0.001;
x_k_1(1) = 2*cos(x_k(5)*dt) * x_k(1) - x_k(2) ;
x_k_1(2) = x_k(1);
x_k_1(3) = 2*cos(x_k(5)*dt) * x_k(3) - x_k(4);
x_k_1(4) = x_k(3);
x_k_1(5) = x_k(5);
 
end

== matlab function quarter_sus_imp_force/QuarterSuspension /Variant Subsystem/Train-Imp_Force/Subsystem/MATLAB Function2/adaptive IFEKF simple/MATLAB Function1 ==
  data: u input; y output
function y = imp_force_filter(u)
    % 声明持久变量，用于保存上一次的输出值
    % 在生成的 C 代码中，这会自动映射为静态变量 (static)
    persistent y_prev
    
    % 定义遗忘因子 (Forgetting Factor)
    % lambda = 0.999 表示保留 99.9% 的历史值
    lambda = 0.999; 
    
    % 初始化逻辑 (仅在模型开始运行时执行一次)
    if isempty(y_prev)
        % 将初始状态设为当前输入值，避免从 0 开始爬升
        y_prev = u;
    end
    
    % 计算指数加权平均
    % 公式: y(k) = lambda * y(k-1) + (1 - lambda) * u(k)
    y = lambda * y_prev + (1 - lambda) * u;
    
    % 更新状态，供下一时刻计算使用
    y_prev = y;
end

== matlab function quarter_sus_imp_force/QuarterSuspension /Variant Subsystem/Train-Imp_Force/Subsystem/MATLAB Function2/adaptive IFEKF simple/MATLAB Function2 ==
  data: u input; y output
function y = imp_force_filter(u)
    % 声明持久变量，用于保存上一次的输出值
    % 在生成的 C 代码中，这会自动映射为静态变量 (static)
    persistent y_prev
    
    % 定义遗忘因子 (Forgetting Factor)
    % lambda = 0.999 表示保留 99.9% 的历史值
    lambda = 0.999; 
    
    % 初始化逻辑 (仅在模型开始运行时执行一次)
    if isempty(y_prev)
        % 将初始状态设为当前输入值，避免从 0 开始爬升
        y_prev = u;
    end
    
    % 计算指数加权平均
    % 公式: y(k) = lambda * y(k-1) + (1 - lambda) * u(k)
    y = lambda * y_prev + (1 - lambda) * u;
    
    % 更新状态，供下一时刻计算使用
    y_prev = y;
end

== matlab function quarter_sus_imp_force/QuarterSuspension /reward_cal/soft_hard_reward_cal1/MATLAB Function ==
  data: susp_deflection input; r_stroke output; max_limit input; weight input; is_violation output; Q_b_deflec input
function [r_stroke, is_violation] = get_barrier_reward(susp_deflection, max_limit, weight,Q_b_deflec)
% GET_BARRIER_REWARD 计算基于对数李雅普诺夫障碍函数(Log-BLF)的悬架行程奖励
% 
% 输入:
%   susp_deflection : 当前悬架动行程 (单位: m, 例如 0.05)
%   max_limit       : 悬架设计的硬限位 (单位: m, 例如 0.08)
%   weight          : 奖励项的权重系数 (通常为正数，例如 1.0 或 10.0)
%
% 输出:
%   r_stroke        : 计算出的奖励值 (负值，越接近限位负得越多)
%   is_violation    : 布尔标志位，如果物理上已经撞击限位返回 true
%
% 数学原理:
%   Barrier Function V(x) = 0.5 * log( x_lim^2 / (x_lim^2 - x^2) )
%   Reward = - weight * V(x)
%
% 注意事项:
%   为了防止 log(0) 或 log(负数) 导致训练中断，代码内部做了软截断处理。

    % 1. 获取绝对值，简化计算
    abs_x = abs(susp_deflection);
    
    % 2. 检查是否发生物理撞击 (仅用于统计或DEBUG)
    if abs_x >= max_limit
        is_violation = true;
    else
        is_violation = false;
    end
    
    % 3. 数值稳定性处理 (Critical for RL)
    % 设定一个安全阈值 epsilon (例如限位的 99% 或 99.9%)
    % 作用：即使 RL 探索时偶尔略微越界，也将其视为"极度接近限位"，
    % 而不是让 log 函数报错。
    safety_margin = 0.999; 
    effective_limit = max_limit * safety_margin;
    
    % 对输入进行截断 (Clamping)
    % 确保计算 log 时，分母永远不会是 0 或负数
    x_clamped = min(abs_x, effective_limit);
    
    % 4. 计算障碍函数值 (BLF)
    % 公式变形：log(A/B) = log(A) - log(B)
    % 这里 A = max_limit^2, B = max_limit^2 - x^2
    % 当 x 接近 max_limit 时，B 接近 0，log(B) 趋向负无穷，
    % V_barrier 趋向正无穷。
    
    numerator = max_limit^2;
    denominator = max_limit^2 - x_clamped^2;
    
    % 计算障碍惩罚 (正值，代表Cost)
    V_barrier = 0.5 * log(numerator / denominator);
    
    % 5. 转化为奖励 (取负)
    r_stroke = -1 * weight * V_barrier;

    % [可选] 极值惩罚增强
    % 如果确实发生了越界(is_violation=true)，可以额外施加一个巨大的阶跃惩罚，
    % 告诉 Agent "这不仅是接近限位，而是已经坏了"。
    if is_violation
        r_stroke = r_stroke + Q_b_deflec; % 额外的硬惩罚，可视情况添加
    end

end

== matlab function quarter_sus_imp_force/QuarterSuspension /reward_cal/reward_cal/cal_reward ==
  data: state_deflec input; b_def input; reward output; Q_flec input
function reward = fun_reward(state_deflec,b_def,Q_flec)

if state_deflec^2 - b_def^2 > -0.0002
    r_dflec = 1000;
else
    r_dflec = 1/2*log(b_def^2/(b_def^2-state_deflec^2));%定义动行程的BLF函数
end
% Q_r = blkdiag(Q,Q_dot);
% state_r  = [state_deflec,acc];
% reward = state * Q * state'+acc * Q_dot * acc'; %简单二次型reward 考虑加速度与四个状态
% reward  = state_r * Q_r * state_r'; %简单二次型 考虑加速度和动行程
reward = r_dflec * Q_flec; % 二次型加BLF组合

== matlab function quarter_sus_imp_force/QuarterSuspension /Variant Subsystem/Vaildation-Force/obsprocess ==
  data: state input; obs output
function obs = fun_done(state)
    obs = zeros(3,1);
    obs_scaling = [1.5, 20, 0.03];
    obs(1) = state(3)/obs_scaling(1);
    obs(2) = state(5)/obs_scaling(2);
    obs(3) = state(6)/obs_scaling(3);
%     for t=7:1:27
%         x = state(1) + delta_t*ref_v*(t-6);
%         obs(t) = ref_A(1)*sin(2*pi/ref_T(1)*x + ref_fai(1)) + ref_A(2)*sin(2*pi/ref_T(2)*x + ref_fai(2)) + ref_A(3)*sin(2*pi/ref_T(3)*x + ref_fai(3));
%     end

end

== matlab function quarter_sus_imp_force/QuarterSuspension /Variant Subsystem/Vaildation-Imp/obsprocess ==
  data: state input; obs output
function obs = fun_done(state)
    obs = zeros(3,1);
    obs_scaling = [1.5, 20, 0.03];
    obs(1) = state(3)/obs_scaling(1);
    obs(2) = state(5)/obs_scaling(2);
    obs(3) = state(6)/obs_scaling(3);
%     for t=7:1:27
%         x = state(1) + delta_t*ref_v*(t-6);
%         obs(t) = ref_A(1)*sin(2*pi/ref_T(1)*x + ref_fai(1)) + ref_A(2)*sin(2*pi/ref_T(2)*x + ref_fai(2)) + ref_A(3)*sin(2*pi/ref_T(3)*x + ref_fai(3));
%     end

end

== matlab function quarter_sus_imp_force/QuarterSuspension /Variant Subsystem/Vaildation-Imp/actprocess ==
  data: act input; real_act output
function real_act = fun_act(act)

real_act= act;
end

== matlab function quarter_sus_imp_force/QuarterSuspension /road_profile/gp/MATLAB Function ==
  data: X input; u output; gp_sample input; x input
function u = u_fn(X, gp_sample, x)
    u = interp1(X, gp_sample, x, 'linear', 'extrap');
end

== stateflow chart quarter_sus_imp_force/QuarterSuspension /Variant Subsystem/Train-Imp_Force/Subsystem/Chart ==
  state L2
    entry:count = 0;
    level = 2;
    during:count = count+1;
    level = 2;
  state L1
    entry:count = 0;
    level = 1;
    during:count = count+1;
    level = 1;
  (default) -> L1
  L1 -> L2 : [freq > (FS1+0.1)&&freq<(FS2-0.1)&&count>=100]
  L2 -> L1 : [(freq<(FS1-0.1)&&count>=100)||(freq>(FS2+0.1)&&count>=100)]
  data: freq input; level output; FS1 input; FS2 input; data local; count local

== matlab function quarter_sus_imp_force/QuarterSuspension /Variant Subsystem/Vaildation-3para-feedback/Subsystem/GOPS_Bridge/actprocess ==
  data: act input; real_act output
function real_act = fun_act(act)

real_act= act;
end

== matlab function quarter_sus_imp_force/QuarterSuspension /Variant Subsystem/Vaildation-3para-feedback/obsprocess ==
  data: state input; obs output
function obs = fun_done(state)
    obs = zeros(3,1);
    obs_scaling = [1.5, 20, 0.03];
    obs(1) = state(3)/obs_scaling(1);
    obs(2) = state(5)/obs_scaling(2);
    obs(3) = state(6)/obs_scaling(3);
%     for t=7:1:27
%         x = state(1) + delta_t*ref_v*(t-6);
%         obs(t) = ref_A(1)*sin(2*pi/ref_T(1)*x + ref_fai(1)) + ref_A(2)*sin(2*pi/ref_T(2)*x + ref_fai(2)) + ref_A(3)*sin(2*pi/ref_T(3)*x + ref_fai(3));
%     end

end
